simulink model "w1p4"  (R2020a)
settings: Solver=VariableStepAuto  StartTime=0.0  StopTime=10.0  RelTol=1e-3
settings Model: Creator=Anjali123  LastModifiedBy=Anjali123

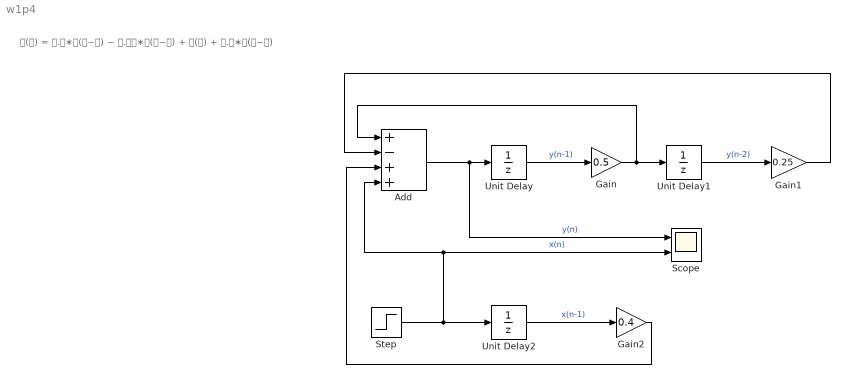
== system w1p4 ==
  note: 𝐲(𝐧) = 𝟎.𝟓∗𝐲(𝐧−𝟏) − 𝟎.𝟐𝟓∗𝐲(𝐧−𝟐) + 𝐱(𝐧) + 𝟎.𝟒∗𝐱(𝐧−𝟏)
  Add : Sum  Inputs=+-++
  Gain : Gain  Gain=0.5
  Gain1 : Gain  Gain=0.25
  Gain2 : Gain  Gain=0.4
  Scope : Scope  NumInputPorts=2
  Step : Step  SampleTime=0.0001
  Unit Delay : UnitDelay  SampleTime=-1  HasFrameUpgradeWarning=on
  Unit Delay1 : UnitDelay  SampleTime=-1  HasFrameUpgradeWarning=on
  Unit Delay2 : UnitDelay  SampleTime=-1  HasFrameUpgradeWarning=on
  wires:
  Unit Delay/1 -> Gain/1  "y(n-1)"
  Add/1 -> Scope/1, Unit Delay/1  "y(n)"
  Unit Delay1/1 -> Gain1/1  "y(n-2)"
  Gain/1 -> Add/1, Unit Delay1/1
  Step/1 -> Scope/2, Add/4, Unit Delay2/1  "x(n)"
  Unit Delay2/1 -> Gain2/1  "x(n-1)"
  Gain1/1 -> Add/2
  Gain2/1 -> Add/3
